simulink model "Difference_Eq"  (R2020b)
settings: Solver=VariableStepAuto  StartTime=0.0  StopTime=10.0  RelTol=1e-3
settings Model: Creator=99003759  LastModifiedBy=99003778

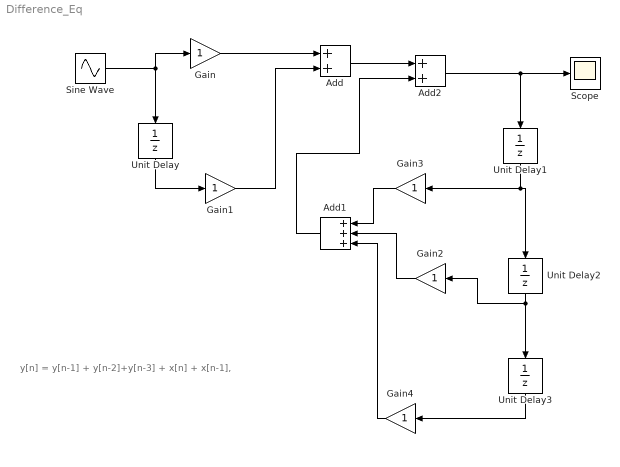
== system Difference_Eq ==
  note: y[n] = y[n-1] + y[n-2]+y[n-3] + x[n] + x[n-1],
  Add : Sum
  Add1 : Sum  Inputs=+++
  Add2 : Sum
  Gain{,1..4} (5 alike) : Gain
  Scope : Scope
  Sine Wave : Sin  SampleTime=0
  Unit Delay{,1..3} (4 alike) : UnitDelay  SampleTime=-1  HasFrameUpgradeWarning=on
  wires:
  Sine Wave/1 -> Unit Delay/1, Gain/1
  Unit Delay/1 -> Gain1/1
  Unit Delay1/1 -> Gain3/1, Unit Delay2/1
  Unit Delay2/1 -> Unit Delay3/1, Gain2/1
  Gain/1 -> Add/1
  Gain1/1 -> Add/2
  Gain3/1 -> Add1/1
  Gain2/1 -> Add1/2
  Add1/1 -> Add2/2
  Add/1 -> Add2/1
  Add2/1 -> Scope/1, Unit Delay1/1
  Unit Delay3/1 -> Gain4/1
  Gain4/1 -> Add1/3
